simulink model "exp10"  (R2025b)
settings: Solver=VariableStepAuto  StartTime=0.0  StopTime=10.0  RelTol=1e-3
libraries: simulink_extras x5
settings Model: Creator=shanm  LastModifiedBy=SUBHASH

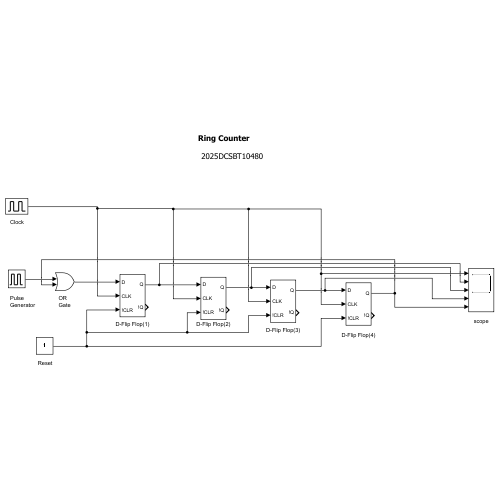
[thumbnail: Simulink's stored preview of the top-level diagram]
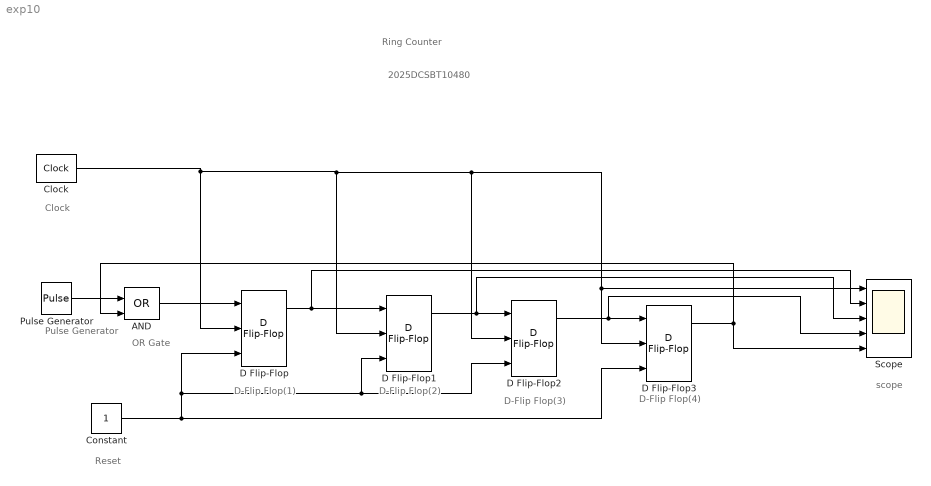
== system exp10 ==
  note: D-Flip Flop(1)
  note: Clock
  note: 2025DCSBT10480
  note: Ring Counter
  note: Pulse
      | Generator
  note: Reset
  note: OR
      | Gate
  note: D-Flip Flop(2)
  note: D-Flip Flop(3)
  note: D-Flip Flop(4)
  note: scope
  AND : Logic  Operator=OR  IconShape=distinctive  AllPortsSameDT=off  OutDataTypeStr=boolean
  Clock : simulink_extras/Flip Flops/Clock  period=2
  Constant : Constant
  D Flip-Flop{,1..3} (4 alike) : simulink_extras/Flip Flops/D Flip-Flop
  Pulse Generator : DiscretePulseGenerator  PulseType=Time based  Period=10  PulseWidth=30
  Scope : Scope  NumInputPorts=5
      settings: ActiveDisplayYMinimum=-0.12499999999999997  ActiveDisplayYMaximum=1.125
  wires:
  Pulse Generator/1 -> AND/1
  D Flip-Flop/1 -> Scope/2, D Flip-Flop1/1
  D Flip-Flop1/1 -> Scope/3, D Flip-Flop2/1
  D Flip-Flop2/1 -> Scope/4, D Flip-Flop3/1
  Clock/1 -> Scope/1, D Flip-Flop3/2, D Flip-Flop2/2, D Flip-Flop1/2, D Flip-Flop/2
  D Flip-Flop3/1 -> AND/2, Scope/5
  AND/1 -> D Flip-Flop/1
  Constant/1 -> D Flip-Flop3/3, D Flip-Flop1/3, D Flip-Flop2/3, D Flip-Flop/3
